simulink model "Proyecto_CyS_SILVA"  (R2019a)
settings: Solver=VariableStepAuto  StartTime=0.0  StopTime=10.0  MaxStep=1e-4  RelTol=1e-3
undefined symbols (not defined in the file): A, B, Bd, C, K, kr, L, r, sigbuilder_block, Tl, Va, x0
libraries: commchan3 x1
settings Model: Creator=Víctor  LastModifiedBy=Víctor

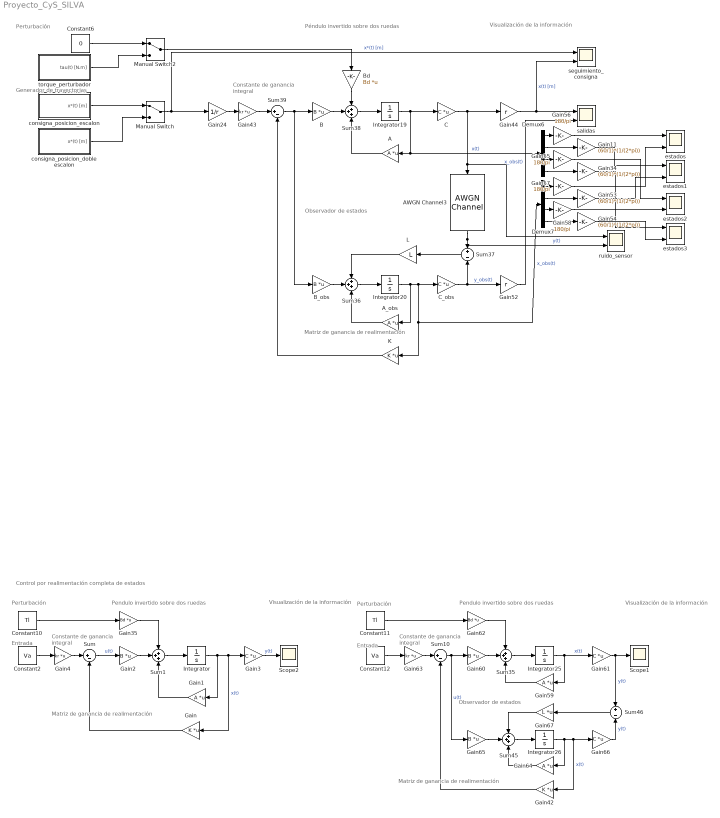
== system Proyecto_CyS_SILVA ==
  note: Generador de trayectorias
  note: Perturbación
  note: Péndulo invertido sobre dos ruedas
  note: Observador de estados
  note: Matriz de ganancia de
      | realimentación
  note: Visualización de la información
  note: Constante de
      | ganancia integral
  note: Matriz de ganancia de realimentación
  note: Observador de estados
  note: Constante de
      | ganancia integral
  note: Visualización de
      | la información
  note: Entrada
  note: Control por realimentación completa de estados
  note: Pendulo invertido sobre dos ruedas
  note: Entrada
  note: Matriz de ganancia de realimentación
  note: Perturbación
  note: Pendulo invertido sobre dos ruedas
  note: Perturbación
  note: Constante de
      | ganancia integral
  note: Visualización de
      | la información
  A : Gain  Gain=A  Multiplication=Matrix(K*u)
  AWGN Channel3 : commchan3/AWGN Channel  InputProcessing=Columns as channels (frame based)  seed=67  noiseMode=Variance from mask  EbNodB=10  EsNodB=10  SNRdB=10  bitsPerSym=1  Ps=1  Tsym=1  variance=var
      settings: SourceProductName=Communications Toolbox
  A_obs : Gain  Gain=A  Multiplication=Matrix(K*u)
  B : Gain  Gain=B  Multiplication=Matrix(K*u)
  B_obs : Gain  Gain=B  Multiplication=Matrix(K*u)
  Bd : Gain  Gain=Bd  Multiplication=Matrix(K*u)
  C : Gain  Gain=C  Multiplication=Matrix(K*u)
  C_obs : Gain  Gain=C  Multiplication=Matrix(K*u)
  Constant10 : Constant  Value=Tl
  Constant11 : Constant  Value=Tl
  Constant12 : Constant  Value=Va
  Constant2 : Constant  Value=Va
  Constant6 : Constant  Value=0
  Demux6 : Demux
  Demux7 : Demux
  Gain : Gain  Gain=K  Multiplication=Matrix(K*u)
  Gain1 : Gain  Gain=A  Multiplication=Matrix(K*u)
  Gain{11,34,53..54} (4 alike) : Gain  Gain=(60/1)*(1/(2*pi))
  Gain2 : Gain  Gain=B  Multiplication=Matrix(K*u)
  Gain24 : Gain  Gain=1/r
  Gain3 : Gain  Gain=C  Multiplication=Matrix(K*u)
  Gain35 : Gain  Gain=Bd  Multiplication=Matrix(K*u)
  Gain4 : Gain  Gain=kr  Multiplication=Matrix(K*u)
  Gain42 : Gain  Gain=K  Multiplication=Matrix(K*u)
  Gain43 : Gain  Gain=kr  Multiplication=Matrix(K*u)
  Gain44 : Gain  Gain=r
  Gain52 : Gain  Gain=r
  Gain{55..58} (4 alike) : Gain  Gain=180/pi
  Gain59 : Gain  Gain=A  Multiplication=Matrix(K*u)
  Gain60 : Gain  Gain=B  Multiplication=Matrix(K*u)
  Gain61 : Gain  Gain=C  Multiplication=Matrix(K*u)
  Gain62 : Gain  Gain=Bd  Multiplication=Matrix(K*u)
  Gain63 : Gain  Gain=kr  Multiplication=Matrix(K*u)
  Gain64 : Gain  Gain=A  Multiplication=Matrix(K*u)
  Gain65 : Gain  Gain=B  Multiplication=Matrix(K*u)
  Gain66 : Gain  Gain=C  Multiplication=Matrix(K*u)
  Gain67 : Gain  Gain=L  Multiplication=Matrix(K*u)
  Integrator{,19..20,25..26} (5 alike) : Integrator  InitialCondition=x0
  K : Gain  Gain=K  Multiplication=Matrix(K*u)
  L : Gain  Gain=L
  Manual Switch : ManualSwitch
  Manual Switch2 : ManualSwitch
  Scope1 : Scope
  Scope2 : Scope
  Sum : Sum  Inputs=|+-
  Sum{1,35..36,38,45} (5 alike) : Sum  Inputs=+++
  Sum10 : Sum  Inputs=|+-
  Sum37 : Sum  Inputs=+-
  Sum39 : Sum  Inputs=|+-
  Sum46 : Sum  Inputs=+-
  consigna_posicion_doble escalon : Subsystem  Tag=STV Subsys  LoadFcn=sigbuilder_block('load');  StartFcn=sigbuilder_block('start');  StopFcn=sigbuilder_block('stop');  ClipboardFcn=sigbuilder_block('clipboard');  mask(Sigbuilder block){tuvar=[0:10]}
      mask help: Simulink:masks:SigbuilderBlock_MD
      mask init:
      | if ~strcmp(get_param(bdroot(gcbh),'SimulationStatus'),'stopped') tuvar = sigbuilder_block('maskInit'); end
      settings: CopyFcn=sigbuilder_block('copy');  DeleteFcn=sigbuilder_block('delete');  ModelCloseFcn=sigbuilder_block('modelClose');  PreSaveFcn=sigbuilder_block('preSave');  PauseFcn=sigbuilder_block('pause');  ContinueFcn=sigbuilder_block('continue');  NameChangeFcn=sigbuilder_block('namechange');  OpenFcn=sigbuilder_block('open',[437.6 153 550.4 359.25 ]);  CloseFcn=sigbuilder_block('close');
      mask Display: plot(0, 0, 100, 100,[2, 2, 32, 32, 2], [68, 8, 8, 68, 68],[32, 2], [38, 38], [32, 19, 2],[53, 60, 44], [32, 17, 17, 2],[16, 16, 31, 31]);txt = getActiveGroup(gcbh);text(2, 100, txt,'verticalAlignment', 'top');
  consigna_posicion_escalon : Subsystem  Tag=STV Subsys  LoadFcn=sigbuilder_block('load');  StartFcn=sigbuilder_block('start');  StopFcn=sigbuilder_block('stop');  ClipboardFcn=sigbuilder_block('clipboard');  mask(Sigbuilder block){tuvar=[0:10]}
      mask help: Simulink:masks:SigbuilderBlock_MD
      mask init:
      | if ~strcmp(get_param(bdroot(gcbh),'SimulationStatus'),'stopped') tuvar = sigbuilder_block('maskInit'); end
      settings: CopyFcn=sigbuilder_block('copy');  DeleteFcn=sigbuilder_block('delete');  ModelCloseFcn=sigbuilder_block('modelClose');  PreSaveFcn=sigbuilder_block('preSave');  PauseFcn=sigbuilder_block('pause');  ContinueFcn=sigbuilder_block('continue');  NameChangeFcn=sigbuilder_block('namechange');  OpenFcn=sigbuilder_block('open',[437.6 153 550.4 359.25 ]);  CloseFcn=sigbuilder_block('close');
      mask Display: plot(0, 0, 100, 100,[2, 2, 32, 32, 2], [68, 8, 8, 68, 68],[32, 2], [38, 38], [32, 19, 2],[53, 60, 44], [32, 17, 17, 2],[16, 16, 31, 31]);txt = getActiveGroup(gcbh);text(2, 100, txt,'verticalAlignment', 'top');
  estados{,1..3} (4 alike) : Scope  NumInputPorts=2
  ruido_sensor : Scope  NumInputPorts=2
  salidas : Scope  NumInputPorts=2
  seguimiento_consigna : Scope  NumInputPorts=2
  torque_perturbador : Subsystem  Tag=STV Subsys  LoadFcn=sigbuilder_block('load');  StartFcn=sigbuilder_block('start');  StopFcn=sigbuilder_block('stop');  ClipboardFcn=sigbuilder_block('clipboard');  mask(Sigbuilder block){tuvar=[0:10]}
      mask help: Simulink:masks:SigbuilderBlock_MD
      mask init:
      | if ~strcmp(get_param(bdroot(gcbh),'SimulationStatus'),'stopped') tuvar = sigbuilder_block('maskInit'); end
      settings: CopyFcn=sigbuilder_block('copy');  DeleteFcn=sigbuilder_block('delete');  ModelCloseFcn=sigbuilder_block('modelClose');  PreSaveFcn=sigbuilder_block('preSave');  PauseFcn=sigbuilder_block('pause');  ContinueFcn=sigbuilder_block('continue');  NameChangeFcn=sigbuilder_block('namechange');  OpenFcn=sigbuilder_block('open',[437.6 153 550.4 359.25 ]);  CloseFcn=sigbuilder_block('close');
      mask Display: plot(0, 0, 100, 100,[2, 2, 32, 32, 2], [68, 8, 8, 68, 68],[32, 2], [38, 38], [32, 19, 2],[53, 60, 44], [32, 17, 17, 2],[16, 16, 31, 31]);txt = getActiveGroup(gcbh);text(2, 100, txt,'verticalAlignment', 'top');
  wires:
  Gain57/1 -> estados/2
  C_obs/1 -> Gain52/1, Sum37/2  "y_obs(t)"
  consigna_posicion_doble escalon/1(x*(t) [m]) -> Manual Switch/2
  Demux7/2 -> Gain53/1
  Demux7/3 -> Gain58/1
  Gain56/1 -> estados/1
  Demux6/1 -> Gain56/1
  Demux7/4 -> Gain54/1
  Demux7/1 -> Gain57/1
  Gain11/1 -> estados1/1
  Gain58/1 -> estados2/2
  Gain55/1 -> estados2/1
  Demux6/4 -> Gain34/1
  Demux6/2 -> Gain11/1
  Gain52/1 -> salidas/2  "x_obs(t)"
  Bd/1 -> Sum38/1
  A/1 -> Sum38/3
  Gain54/1 -> estados3/2
  consigna_posicion_escalon/1(x*(t) [m]) -> Manual Switch/1
  torque_perturbador/1(tau(t) [N.m]) -> Manual Switch2/2
  C/1 -> ruido_sensor/1, AWGN Channel3/1, Gain44/1  "y(t)"
  Manual Switch/1 -> seguimiento_consigna/1, Gain24/1  "x*(t) [m]"
  AWGN Channel3/1 -> Sum37/1, ruido_sensor/2
  Constant6/1 -> Manual Switch2/1
  Gain34/1 -> estados3/1
  Gain53/1 -> estados1/2
  Integrator19/1 -> Demux6/1, A/1, C/1  "x(t)"
  A_obs/1 -> Sum36/3
  Manual Switch2/1 -> Bd/1
  Gain43/1 -> Sum39/1
  L/1 -> Sum36/1
  Sum36/1 -> Integrator20/1
  Sum38/1 -> Integrator19/1
  B/1 -> Sum38/2
  K/1 -> Sum39/2
  Integrator20/1 -> C_obs/1, Demux7/1, K/1, A_obs/1  "x_obs(t)"
  B_obs/1 -> Sum36/2
  Sum39/1 -> B_obs/1, B/1
  Gain44/1 -> seguimiento_consigna/2, salidas/1  "x(t) [m]"
  Demux6/3 -> Gain55/1
  Gain24/1 -> Gain43/1
  Sum37/1 -> L/1
  Gain2/1 -> Sum1/2
  Integrator25/1 -> Gain61/1, Gain59/1  "x(t)"
  Integrator/1 -> Gain1/1, Gain/1, Gain3/1  "x(t)"
  Gain66/1 -> Sum46/2  "y(t)"
  Gain65/1 -> Sum45/2
  Gain67/1 -> Sum45/1
  Sum35/1 -> Integrator25/1
  Integrator26/1 -> Gain64/1, Gain42/1, Gain66/1  "x(t)"
  Gain61/1 -> Sum46/1, Scope1/1  "y(t)"
  Sum10/1 -> Gain65/1, Gain60/1  "u(t)"
  Constant12/1 -> Gain63/1
  Constant10/1 -> Gain35/1
  Gain62/1 -> Sum35/1
  Gain59/1 -> Sum35/3
  Gain1/1 -> Sum1/3
  Gain35/1 -> Sum1/1
  Sum1/1 -> Integrator/1
  Gain63/1 -> Sum10/1
  Gain64/1 -> Sum45/3
  Sum46/1 -> Gain67/1
  Gain3/1 -> Scope2/1  "y(t)"
  Gain/1 -> Sum/2
  Constant11/1 -> Gain62/1
  Gain60/1 -> Sum35/2
  Constant2/1 -> Gain4/1
  Sum/1 -> Gain2/1  "u(t)"
  Gain4/1 -> Sum/1
  Gain42/1 -> Sum10/2
  Sum45/1 -> Integrator26/1

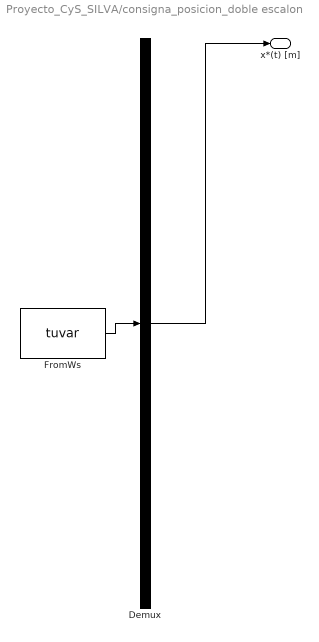
== system Proyecto_CyS_SILVA/consigna_posicion_doble escalon ==
  Demux : Demux  Tag=STV Demux  Outputs=1
  FromWs : FromWorkspace  Tag=STV FromWs  VariableName=tuvar  SampleTime=0
      SigBuilderData=|
      | common.afterFinalStr = 'Extrapolate'
      | common.sampleTime = 0
      | dataSet.timeRange = [0 15]
      | dataSet.name = 'Group 1'
      | sbobj.Groups.Name = 'Group 1'
      | sbobj.Groups.Signals.Name = 'x*(t) [m]'
      | sbobj.Groups.Signals.XData = [0 1 2 2 6 6 8 15]
      | sbobj.Groups.Signals.YData = [0 0 0 1 1 -1 -1 -1]
      | sbobj.Groups.TimeRange = [0 15]
  x*(t) [m] : Outport  Tag=STV Outport
  wires:
  Demux/1 -> x*(t) [m]/1
  FromWs/1 -> Demux/1

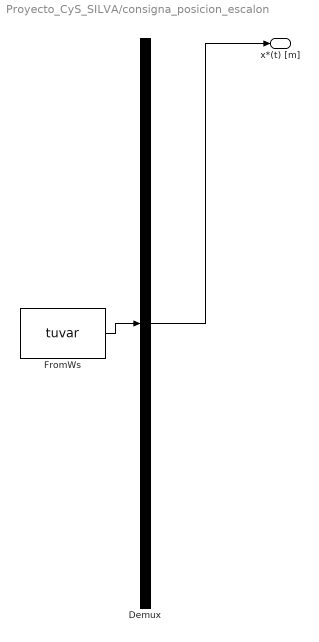
== system Proyecto_CyS_SILVA/consigna_posicion_escalon ==
  Demux : Demux  Tag=STV Demux  Outputs=1
  FromWs : FromWorkspace  Tag=STV FromWs  VariableName=tuvar  SampleTime=0
      SigBuilderData=|
      | common.afterFinalStr = 'Extrapolate'
      | common.sampleTime = 0
      | dataSet.timeRange = [0 15]
      | dataSet.name = 'Group 1'
      | sbobj.Groups.Name = 'Group 1'
      | sbobj.Groups.Signals.Name = 'x*(t) [m]'
      | sbobj.Groups.Signals.XData = [0 1 2 2 6 8 15]
      | sbobj.Groups.Signals.YData = [0 0 0 1 1 1 1]
      | sbobj.Groups.TimeRange = [0 15]
  x*(t) [m] : Outport  Tag=STV Outport
  wires:
  FromWs/1 -> Demux/1
  Demux/1 -> x*(t) [m]/1

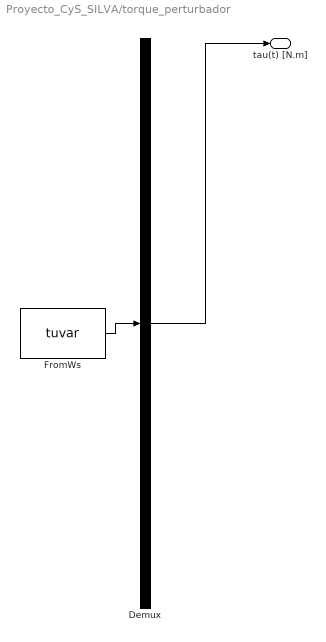
== system Proyecto_CyS_SILVA/torque_perturbador ==
  Demux : Demux  Tag=STV Demux  Outputs=1
  FromWs : FromWorkspace  Tag=STV FromWs  VariableName=tuvar  SampleTime=0
      SigBuilderData=|
      | common.afterFinalStr = 'Extrapolate'
      | common.sampleTime = 0
      | dataSet.timeRange = [0 15]
      | dataSet.name = 'Group 1'
      | sbobj.Groups.Name = 'Group 1'
      | sbobj.Groups.Signals.Name = 'tau(t) [N.m]'
      | sbobj.Groups.Signals.XData = [0 1 2 6 6 7 7 15]
      | sbobj.Groups.Signals.YData = [0 0 0 0 0.1 0.1 0 0]
      | sbobj.Groups.TimeRange = [0 15]
  tau(t) [N.m] : Outport  Tag=STV Outport
  wires:
  FromWs/1 -> Demux/1
  Demux/1 -> tau(t) [N.m]/1
